simulink model "model_shok"  (R2024a)
settings: Solver=VariableStepAuto  StartTime=0.0  StopTime=3  RelTol=1e-8
values from neighbouring files (symbols this model uses):
  B = [0; 4 / (4 * M + m); 0; 3 / (l * (4 * M + m))]    [get_matrices.m]    (also in main.m = [0; 1 / M; 0; 1 / (l * M)])
  C = [1, 0, 0, 0; 0, 0, 1, 0]    [get_matrices.m]    (also in main.m)
  Gl = [-5, 1; 0, -5]    [chapter3.m]    (also in main.m)
  K = Y / P    [TAU.m]    (also in chapter3.m = TAU.FindControllerSylvester(A, B, GammaK); chapter4.m = pairs{i}{1}; chapter6.m = TAU.FindControllerLMI(A, B, 2); main.m = FindControllerSylvester(A, B, GammaK))
  l = l / 2    [get_initials.m]    (also in main.m)
  M = randi([100000 1000000]) / 1000 / sqrt(2)    [get_initials.m]    (also in main.m)
  m = randi([1000 10000]) / 1000 * sqrt(3)    [get_initials.m]    (also in main.m)
  theta0 = 0.1    [chapter2.m]    (also in chapter3.m; chapter4.m = 0.2; chapter5.m = 0.2; chapter6.m = 0.2)
undefined symbols (not defined in the file or in its folder): Ql, Yl
settings Model: Creator=alexivanov  LastModifiedBy=alexivanov

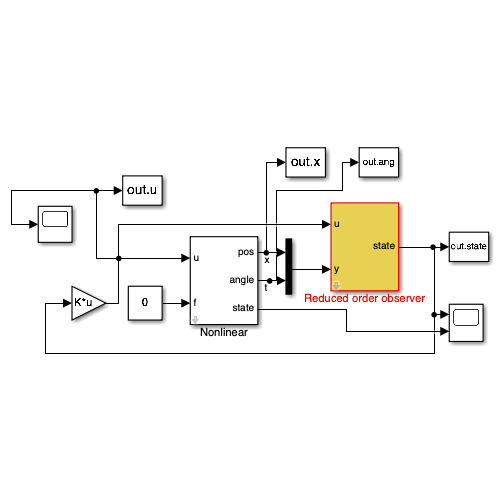
[thumbnail: Simulink's stored preview of the top-level diagram]
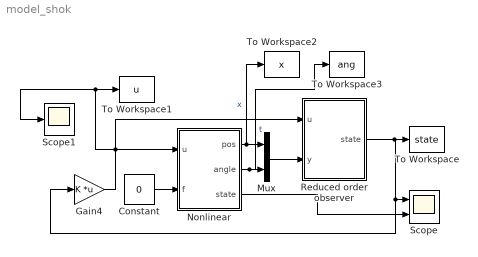
== system model_shok ==
  Constant : Constant  Value=0
  Gain4 : Gain  Gain=K  Multiplication=Matrix(K*u)
  Mux : Mux  Inputs=2
  Nonlinear : Subsystem  mask{Mcart=M, m=m, l=l, g=9.81, theta0=theta0}
      mask prompts: Mcart "Mass of cart (kg)"; m "Mass of pend (kg)"; l "Length of pend (m)"; theta0 "Initial angle (rad)"
  Reduced order observer : Subsystem  mask{Mcart=M, m=m, l=l, g=9.81, theta0=theta0}
      mask prompts: Mcart "Mass of cart (kg)"; m "Mass of pend (kg)"; l "Length of pend (m)"; theta0 "Initial angle (rad)"
  Scope : Scope  NumInputPorts=2
  Scope1 : Scope
  To Workspace : ToWorkspace  VariableName=state  SampleTime=-1
  To Workspace1 : ToWorkspace  VariableName=u  SampleTime=-1
  To Workspace2 : ToWorkspace  VariableName=x  SampleTime=-1
  To Workspace3 : ToWorkspace  VariableName=ang  SampleTime=-1
  wires:
  Gain4/1 -> Nonlinear/1(u), Scope1/1, To Workspace1/1, Reduced order observer/1(u)
  Nonlinear/2(angle) -> To Workspace3/1, Mux/2  "t"
  Mux/1 -> Reduced order observer/2(y)
  Nonlinear/1(pos) -> To Workspace2/1, Mux/1  "x"
  Constant/1 -> Nonlinear/2(f)
  Reduced order observer/1(state) -> Gain4/1, Scope/1, To Workspace/1
  Nonlinear/3(state) -> Scope/2

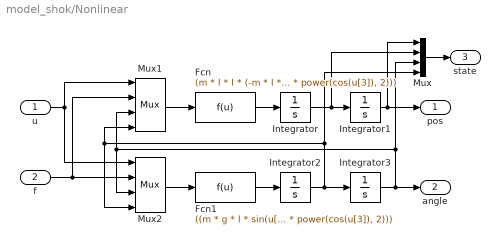
== system model_shok/Nonlinear ==
  u : Inport
  f : Inport  Port=2
  Fcn : Fcn  Expr=(m * l * l * (-m * l * power(u[4], 2) * sin(u[3]) + u[1]) + m * l * cos(u[3]) * (m * g * l * sin(u[3]) + u[2])) / (m * l * l * (Mcart + m - m * power(cos(u[3]), 2)))
  Fcn1 : Fcn  Expr=((m * g * l * sin(u[3]) + u[2]) * (Mcart + m) + m * l * cos(u[3]) * (-m * l * power(u[4], 2) * sin(u[3]) + u[1])) / (m * l * l * (Mcart + m - m * power(cos(u[3]), 2)))
  Integrator : Integrator
  Integrator1 : Integrator
  Integrator2 : Integrator
  Integrator3 : Integrator  InitialCondition=theta0
  Mux : Mux
  Mux1 : Mux
  Mux2 : Mux
  pos : Outport
  angle : Outport  Port=2
  state : Outport  Port=3
  wires:
  Integrator1/1 -> Mux/1, pos/1
  Integrator/1 -> Mux/2, Integrator1/1
  Integrator2/1 -> Mux/4, Mux1/4, Mux2/4, Integrator3/1
  Integrator3/1 -> Mux/3, Mux2/3, Mux1/3, angle/1
  Fcn/1 -> Integrator/1
  u/1 -> Mux2/1, Mux1/1
  f/1 -> Mux2/2, Mux1/2
  Fcn1/1 -> Integrator2/1
  Mux2/1 -> Fcn1/1
  Mux1/1 -> Fcn/1
  Mux/1 -> state/1

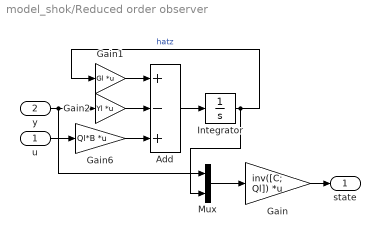
== system model_shok/Reduced order observer ==
  u : Inport
  y : Inport  Port=2
  Add : Sum  Inputs=+-+
  Gain : Gain  Gain=inv([C; Ql])  Multiplication=Matrix(K*u)
  Gain1 : Gain  Gain=Gl  Multiplication=Matrix(K*u)
  Gain2 : Gain  Gain=Yl  Multiplication=Matrix(K*u)
  Gain6 : Gain  Gain=Ql*B  Multiplication=Matrix(K*u)
  Integrator : Integrator
  Mux : Mux  Inputs=2
  state : Outport
  wires:
  Add/1 -> Integrator/1
  Gain1/1 -> Add/1
  Integrator/1 -> Gain1/1, Mux/2  "hatz"
  y/1 -> Mux/1, Gain2/1
  Gain2/1 -> Add/2
  u/1 -> Gain6/1
  Gain6/1 -> Add/3
  Mux/1 -> Gain/1
  Gain/1 -> state/1
